simulink model "Inner2"  (Simulink 5.0)
settings: Solver=ode45  StartTime=0.0  StopTime=10.0  RelTol=1e-3
undefined symbols (not defined in the file): sigbuilder_block
settings Model: Creator=scaife  LastModifiedBy=scaife  ExtModeAutoUpdateStatusClock=off

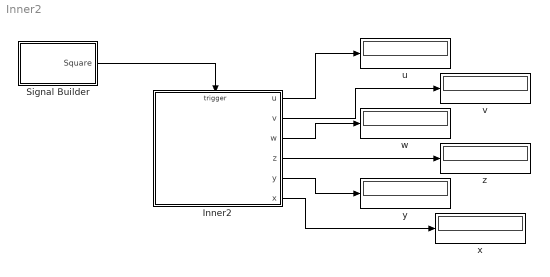
== system Inner2 ==
  Inner2 : Stateflow chart
  Signal Builder : Subsystem  Tag=STV Subsys  StartFcn=sigbuilder_block('start');  StopFcn=sigbuilder_block('stop');  ClipboardFcn=sigbuilder_block('clipboard');  mask(Sigbuilder block){}
      mask help: Sigbuilder GUI
      mask init:
      | if ~strcmp(get_param(bdroot(gcb),'SimulationStatus'),'stopped') tuvar = sigbuilder_block('maskInit'); end
      settings: CopyFcn=sigbuilder_block('copy');  DeleteFcn=sigbuilder_block('delete');  ModelCloseFcn=sigbuilder_block('modelClose');  PreSaveFcn=sigbuilder_block('preSave');  NameChangeFcn=sigbuilder_block('namechange');  OpenFcn=sigbuilder_block('open',[50 50 520 400 ]);  CloseFcn=sigbuilder_block('close');
      mask Display: plot(0,0,100,100,[10,10,40,40,10],[80,20,20,80,80],[40,10],[50,50], [40,27,10],[65,72,56],[40,25,25,10],[28,28,43,43]);
  u : Display
  v : Display
  w : Display
  x : Display
  y : Display
  z : Display
  wires:
  Signal Builder/1(Square) -> Inner2/Trigger
  Inner2/1(u) -> u/1
  Inner2/2(v) -> v/1
  Inner2/3(w) -> w/1
  Inner2/4(z) -> z/1
  Inner2/5(y) -> y/1
  Inner2/6(x) -> x/1

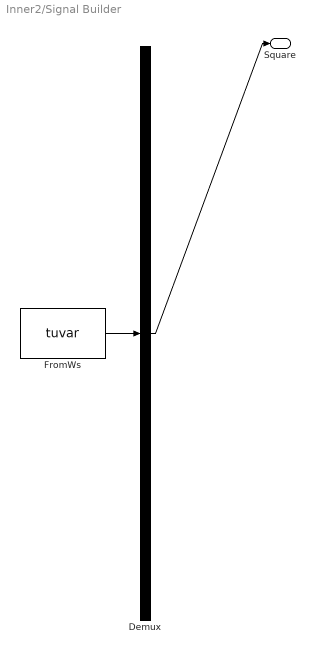
== system Inner2/Signal Builder ==
  Demux : Demux  Tag=STV Demux  Outputs=1
  FromWs : FromWorkspace  Tag=STV FromWs  VariableName=tuvar  SampleTime=0  SigBuilderData=DataTag0
  Square : Outport  Tag=STV Outport
  wires:
  FromWs/1 -> Demux/1
  Demux/1 -> Square/1

== stateflow chart Inner2 ==
  state A/
    en: u+=10000;
    ex: u+=100;
    du: u+=1;
    state A1/
      en: x+=10000;
      ex: x+=100;
      du: x+=1;
    state A2/
      en: v+=10000;
      ex: v+=100;
      du: v+=1;
    A -> A : E[u%%3==0]{w++;}
    A -> A1 : E[u%%3==1]
        | {x+=1000000;}
    A1 -> A : E[u%%3==2]
        | {z++;}
    (default) -> A2 : {v+=1000000;}
  (default) -> A
  data: u output int32; v output int32; w output int32; z output int32; y output int32; x output int32
  events: E input EITHER_EDGE_EVENT
